simulink library "INP_SPDWHL"  (R2024b)
settings: Solver=VariableStepAuto  StartTime=0.0  StopTime=10.0  RelTol=1e-3
libraries: INP_SPDWHL_ManOver x1, INP_SPDWHL_Prep x1
settings Model: Creator=blatak  LastModifiedBy=jmbsp

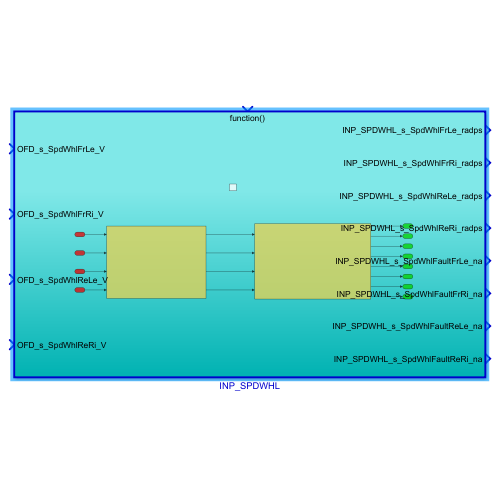
[thumbnail: Simulink's stored preview of the top-level diagram]
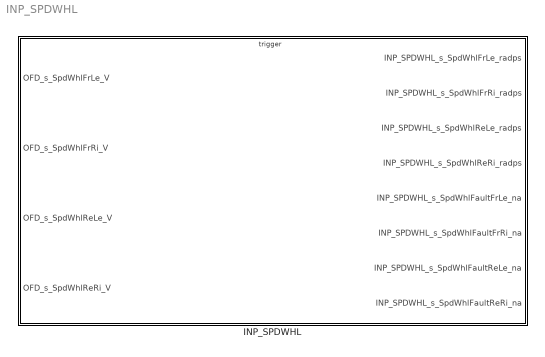
== system INP_SPDWHL ==
  INP_SPDWHL : Subsystem  TreatAsAtomicUnit=on

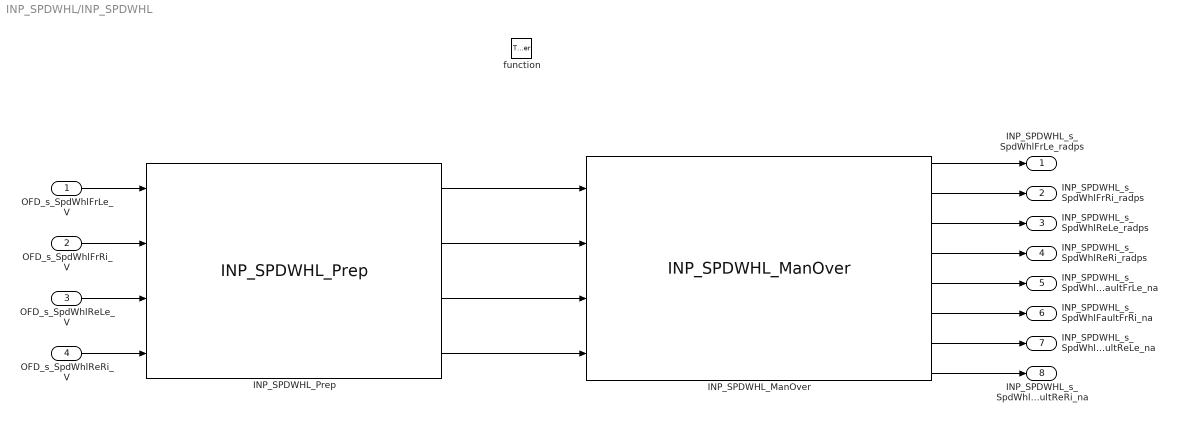
== system INP_SPDWHL/INP_SPDWHL ==
  OFD_s_SpdWhlFrLe_V : Inport
  OFD_s_SpdWhlFrRi_V : Inport  Port=2
  OFD_s_SpdWhlReLe_V : Inport  Port=3
  OFD_s_SpdWhlReRi_V : Inport  Port=4
  function : TriggerPort  TriggerType=function-call  VariantControl=(inherit)
  INP_SPDWHL_ManOver : INP_SPDWHL_ManOver/INP_SPDWHL_ManOver  SystemSampleTime=-1  VariantActivationTime=update diagram  AllowFlexibleInterface=on  Latency=0  AutoFrameSizeCalculation=off
  INP_SPDWHL_Prep : INP_SPDWHL_Prep/INP_SPDWHL_Prep  SystemSampleTime=-1  VariantActivationTime=update diagram  AllowFlexibleInterface=on  Latency=0  AutoFrameSizeCalculation=off
  INP_SPDWHL_s_SpdWhlFrLe_radps : Outport
  INP_SPDWHL_s_SpdWhlFrRi_radps : Outport  Port=2
  INP_SPDWHL_s_SpdWhlReLe_radps : Outport  Port=3
  INP_SPDWHL_s_SpdWhlReRi_radps : Outport  Port=4
  INP_SPDWHL_s_SpdWhlFaultFrLe_na : Outport  Port=5
  INP_SPDWHL_s_SpdWhlFaultFrRi_na : Outport  Port=6
  INP_SPDWHL_s_SpdWhlFaultReLe_na : Outport  Port=7
  INP_SPDWHL_s_SpdWhlFaultReRi_na : Outport  Port=8
  wires:
  INP_SPDWHL_Prep/1 -> INP_SPDWHL_ManOver/1
  INP_SPDWHL_Prep/2 -> INP_SPDWHL_ManOver/2
  INP_SPDWHL_Prep/3 -> INP_SPDWHL_ManOver/3
  INP_SPDWHL_Prep/4 -> INP_SPDWHL_ManOver/4
  OFD_s_SpdWhlFrLe_V/1 -> INP_SPDWHL_Prep/1
  OFD_s_SpdWhlFrRi_V/1 -> INP_SPDWHL_Prep/2
  OFD_s_SpdWhlReLe_V/1 -> INP_SPDWHL_Prep/3
  OFD_s_SpdWhlReRi_V/1 -> INP_SPDWHL_Prep/4
  INP_SPDWHL_ManOver/1 -> INP_SPDWHL_s_SpdWhlFrLe_radps/1
  INP_SPDWHL_ManOver/2 -> INP_SPDWHL_s_SpdWhlFrRi_radps/1
  INP_SPDWHL_ManOver/3 -> INP_SPDWHL_s_SpdWhlReLe_radps/1
  INP_SPDWHL_ManOver/4 -> INP_SPDWHL_s_SpdWhlReRi_radps/1
  INP_SPDWHL_ManOver/5 -> INP_SPDWHL_s_SpdWhlFaultFrLe_na/1
  INP_SPDWHL_ManOver/6 -> INP_SPDWHL_s_SpdWhlFaultFrRi_na/1
  INP_SPDWHL_ManOver/7 -> INP_SPDWHL_s_SpdWhlFaultReLe_na/1
  INP_SPDWHL_ManOver/8 -> INP_SPDWHL_s_SpdWhlFaultReRi_na/1
